simulink model "System_Model_discrete"  (Simulink 7.6)
settings: Solver=ode15s  StartTime=0.0  StopTime=3  RelTol=1e-3
undefined symbols (not defined in the file): C, dd, denhigh, denlow, DiscIntNeverNeededParam, F, G, g, H, K, L0, m, magnitude, nd, Nu, numhigh, numlow, Nx, Q, R, Ts, u0, x01, x02, x03
libraries: fl_lib x18, nesl_utility x6, simulink x5, elec_lib x1
CloseFcn:
  | rtwprivate ssgencode ModelCloseRequest System_Model1
settings Model: Creator=Fodi  LastModifiedBy=Fodi

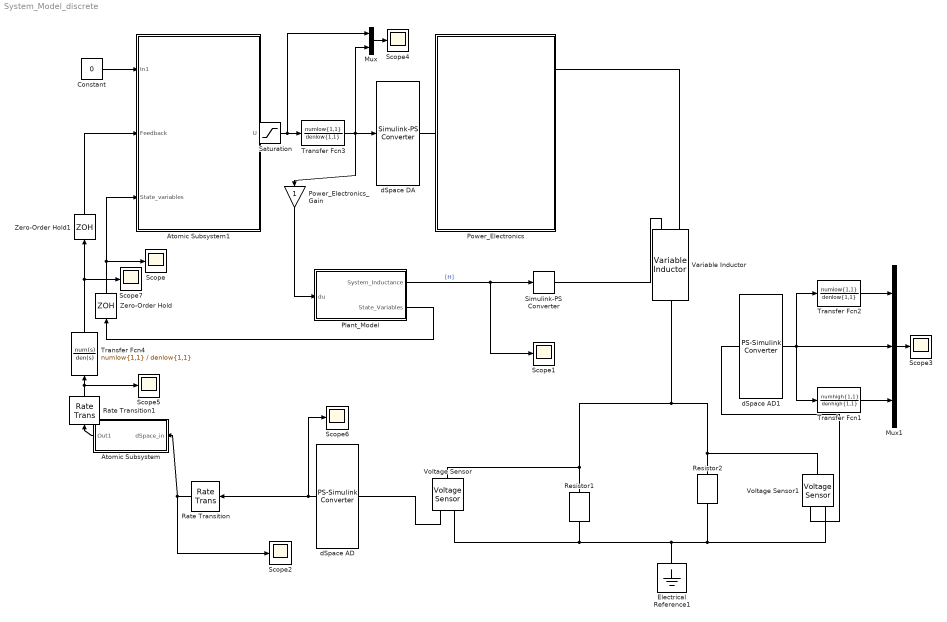
== system System_Model_discrete ==
  Atomic Subsystem : Subsystem  TreatAsAtomicUnit=on
  Atomic Subsystem1 : Subsystem  TreatAsAtomicUnit=on  SystemSampleTime=Ts
  Constant : Constant  Value=0
  Electrical Reference1 : fl_lib/Electrical/Electrical Elements/Electrical Reference  DialogController=NetworkEngine.DynNeDlgSource  SystemSampleTime=-1  i_Log=off  LocalVarNames=|i  LocalVarDescs=|i  LocalVarLogging=0
  Mux : Mux  Inputs=2
  Mux1 : Mux  Inputs=3
  Plant_Model : Subsystem
  Power_Electronics : Subsystem
  Power_Electronics_Gain : Gain
  Rate Transition : RateTransition  OutPortSampleTime=0.0001
  Rate Transition1 : RateTransition  OutPortSampleTime=0.0001
  Resistor1 : fl_lib/Electrical/Electrical Elements/Resistor  DialogController=NetworkEngine.DynNeDlgSource  SystemSampleTime=-1  R=100 Ohm  i_Log=off  v_Log=off  LocalVarNames=|i|v  LocalVarDescs=|i|v  LocalVarLogging=[0 0]
  Resistor2 : fl_lib/Electrical/Electrical Elements/Resistor  DialogController=NetworkEngine.DynNeDlgSource  SystemSampleTime=-1  R=100 Ohm  i_Log=off  v_Log=off  LocalVarNames=|i|v  LocalVarDescs=|i|v  LocalVarLogging=[0 0]
  Saturation : Saturate  UpperLimit=3000  LowerLimit=-u0
  Scope{,1..7} (8 alike) : Scope
      Scope settings: YMin=-3e-006  YMax=1.75e-006  SaveName=ScopeData7
      Scope1 settings: YMin=0.266286  YMax=0.266289  SaveName=ScopeData5
      Scope2 settings: YMin=0.266286  YMax=0.266289  SaveName=ScopeData4
      Scope3 settings: YMin=-2.5  YMax=50  SaveName=ScopeData10
      Scope4 settings: YMin=0.1375  YMax=0.142  SaveName=ScopeData6
      Scope5 settings: YMin=0.266286  YMax=0.266289  SaveName=ScopeData11
      Scope6 settings: TimeRange=0.0315055374939181  YMin=-25.11022062082716  YMax=-22.69283608820259  SaveName=ScopeData12
      Scope7 settings: YMin=0.266286  YMax=0.266289  SaveName=ScopeData20
  Simulink-PS Converter : nesl_utility/Simulink-PS Converter  DialogController=NetworkEngine.DynNeUtilDlgSource  SystemSampleTime=-1  PhysicalDomain=network_engine_domain  LeftPortType=input  RightPortType=output  SubClassName=ps_input  Unit=1  AffineConversion=off  InputFilterTimeConstant=.001  UdotUserProvided=0
  Transfer Fcn1 : TransferFcn  Numerator=numhigh{1,1}  Denominator=denhigh{1,1}
  Transfer Fcn2 : TransferFcn  Numerator=numlow{1,1}  Denominator=denlow{1,1}
  Transfer Fcn3 : TransferFcn  Numerator=numlow{1,1}  Denominator=denlow{1,1}
  Transfer Fcn4 : TransferFcn  Numerator=numlow{1,1}  Denominator=denlow{1,1}
  Variable Inductor : elec_lib/Passive Devices/Variable Inductor  DialogController=NetworkEngine.DynNeDlgSource  SystemSampleTime=-1  prm=2  Lmin=1e-6 H  g=1e-9 1/Ohm  i0=0 A  phi0=0 Wb  LocalVarLogging=[]
  Voltage Sensor : fl_lib/Electrical/Electrical Sensors/Voltage Sensor  DialogController=NetworkEngine.DynNeDlgSource  SystemSampleTime=-1  i1_Log=off  v1_Log=off  LocalVarNames=|i1|v1  LocalVarDescs=|i1|v1  LocalVarLogging=[0 0]
  Voltage Sensor1 : fl_lib/Electrical/Electrical Sensors/Voltage Sensor  DialogController=NetworkEngine.DynNeDlgSource  SystemSampleTime=-1  i1_Log=off  v1_Log=off  LocalVarNames=|i1|v1  LocalVarDescs=|i1|v1  LocalVarLogging=[0 0]
  Zero-Order Hold : ZeroOrderHold  SampleTime=Ts
  Zero-Order Hold1 : ZeroOrderHold  SampleTime=0.001
  dSpace AD : nesl_utility/PS-Simulink Converter  DialogController=NetworkEngine.DynNeUtilDlgSource  SystemSampleTime=-1  PhysicalDomain=network_engine_domain  LeftPortType=input  RightPortType=output  SubClassName=ps_output  Unit=1  AffineConversion=off
  dSpace AD1 : nesl_utility/PS-Simulink Converter  DialogController=NetworkEngine.DynNeUtilDlgSource  SystemSampleTime=-1  PhysicalDomain=network_engine_domain  LeftPortType=input  RightPortType=output  SubClassName=ps_output  Unit=1  AffineConversion=off
  dSpace DA : nesl_utility/Simulink-PS Converter  DialogController=NetworkEngine.DynNeUtilDlgSource  SystemSampleTime=-1  PhysicalDomain=network_engine_domain  LeftPortType=input  RightPortType=output  SubClassName=ps_input  Unit=1  AffineConversion=off  InputFilterTimeConstant=.001  UdotUserProvided=0
  wires:
  Plant_Model/1(System_Inductance) -> Scope1/1, Simulink-PS Converter/1  "[H]"
  Atomic Subsystem1/1(U) -> Saturation/1
  Power_Electronics_Gain/1 -> Plant_Model/1(du)
  Plant_Model/2(State_Variables) -> Zero-Order Hold/1
  Constant/1 -> Atomic Subsystem1/1(In1)
  dSpace AD/1 -> Rate Transition/1, Scope6/1
  Zero-Order Hold/1 -> Scope/1, Atomic Subsystem1/3(State_variables)
  Rate Transition/1 -> Atomic Subsystem/1(dSpace_in), Scope2/1
  Atomic Subsystem/1(Out1) -> Rate Transition1/1
  Zero-Order Hold1/1 -> Atomic Subsystem1/2(Feedback)
  Saturation/1 -> Mux/1, Transfer Fcn3/1
  Mux/1 -> Scope4/1
  dSpace AD1/1 -> Mux1/2, Transfer Fcn2/1, Transfer Fcn1/1
  Transfer Fcn2/1 -> Mux1/1
  Transfer Fcn1/1 -> Mux1/3
  Mux1/1 -> Scope3/1
  Transfer Fcn3/1 -> dSpace DA/1, Power_Electronics_Gain/1, Mux/2
  Transfer Fcn4/1 -> Zero-Order Hold1/1, Scope7/1
  Rate Transition1/1 -> Scope5/1, Transfer Fcn4/1
  connections:
  dSpace DA/RConn1 -- Power_Electronics/LConn1
  Voltage Sensor/RConn2 -- Resistor2/RConn1 -- Voltage Sensor1/RConn2 -- Electrical Reference1/LConn1 -- Resistor1/RConn1
  Voltage Sensor/RConn1 -- dSpace AD/LConn1
  Simulink-PS Converter/RConn1 -- Variable Inductor/LConn1
  Power_Electronics/RConn1 -- Variable Inductor/LConn2
  Voltage Sensor1/RConn1 -- dSpace AD1/LConn1
  Variable Inductor/RConn1 -- Resistor2/LConn1 -- Voltage Sensor1/LConn1 -- Resistor1/LConn1 -- Voltage Sensor/LConn1

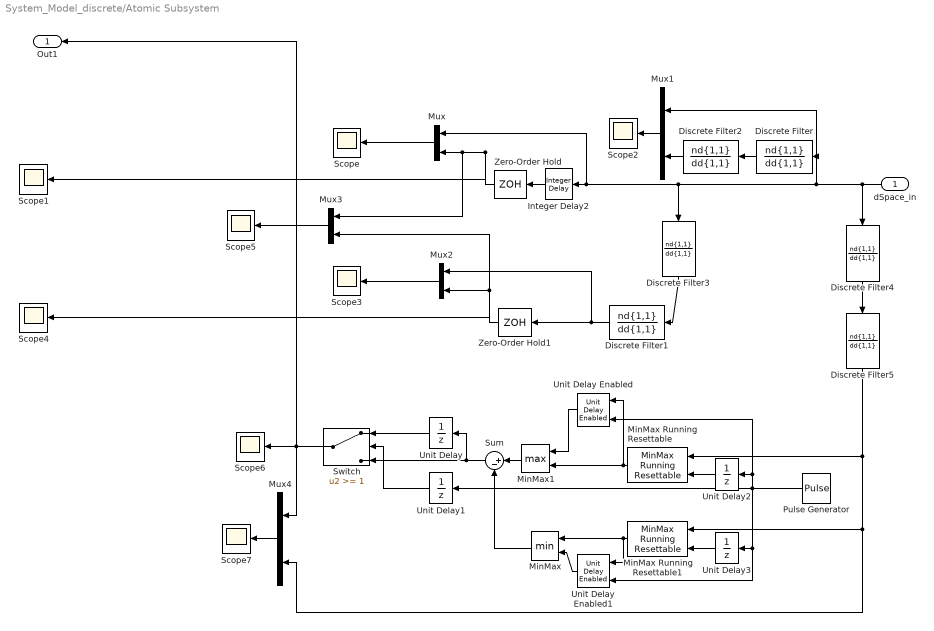
== system System_Model_discrete/Atomic Subsystem ==
  dSpace_in : Inport
  Discrete Filter{,1..5} (6 alike) : DiscreteFilter  Numerator=nd{1,1}  Denominator=dd{1,1}
  Integer Delay2 : simulink/Discrete/Integer Delay  NumDelays=1  vinit=0.0  samptime=-1
  MinMax : MinMax  Inputs=2
  MinMax Running Resettable : simulink/Math Operations/MinMax Running Resettable  SystemSampleTime=-1  Function=max  vinit=0.0
  MinMax Running Resettable1 : simulink/Math Operations/MinMax Running Resettable  SystemSampleTime=-1  Function=min  vinit=0.0
  MinMax1 : MinMax  Function=max  Inputs=2
  Mux{,1..4} (5 alike) : Mux  Inputs=2
  Pulse Generator : DiscretePulseGenerator  Period=10  SampleTime=-1
  Scope{,1..7} (8 alike) : Scope
      Scope settings: TimeRange=7  YMin=-9.407420347240764e-006  YMax=1.255471123145118e-005  SaveName=ScopeData2
      Scope1 settings: TimeRange=7  YMin=-9.407420347240764e-006  YMax=1.255471123145118e-005  SaveName=ScopeData13
      Scope2 settings: TimeRange=7  YMin=-9.407420347240764e-006  YMax=1.255471123145118e-005  SaveName=ScopeData14
      Scope3 settings: TimeRange=7  YMin=-9.407420347240764e-006  YMax=1.255471123145118e-005  SaveName=ScopeData16
      Scope4 settings: TimeRange=7  YMin=-9.407420347240764e-006  YMax=1.255471123145118e-005  SaveName=ScopeData18
      Scope5 settings: TimeRange=7  YMin=-9.407420347240764e-006  YMax=1.255471123145118e-005  SaveName=ScopeData19
      Scope6 settings: TimeRange=3  YMin=0  YMax=1200  SaveName=ScopeData15
      Scope7 settings: TimeRange=7  YMin=-9.407420347240764e-006  YMax=1.255471123145118e-005  SaveName=ScopeData21
  Sum : Sum  Inputs=|+-
  Switch : Switch  Threshold=1
  Unit Delay{,1..3} (4 alike) : UnitDelay  SampleTime=-1
  Unit Delay Enabled : simulink/Additional Math & Discrete/Additional Discrete/Unit Delay Enabled  SystemSampleTime=-1  vinit=0.0  tsamp=-1
  Unit Delay Enabled1 : simulink/Additional Math & Discrete/Additional Discrete/Unit Delay Enabled  SystemSampleTime=-1  vinit=0.0  tsamp=-1
  Zero-Order Hold : ZeroOrderHold  SampleTime=1/1000
  Zero-Order Hold1 : ZeroOrderHold  SampleTime=1/1000
  Out1 : Outport
  wires:
  Zero-Order Hold/1 -> Scope1/1, Mux/2, Mux3/1
  Mux/1 -> Scope/1
  dSpace_in/1 -> Discrete Filter/1, Mux1/1, Mux/1, Integer Delay2/1, Discrete Filter3/1, Discrete Filter4/1
  Integer Delay2/1 -> Zero-Order Hold/1
  Mux1/1 -> Scope2/1
  Discrete Filter/1 -> Discrete Filter2/1
  Zero-Order Hold1/1 -> Scope4/1, Mux2/2, Mux3/2
  Mux2/1 -> Scope3/1
  Discrete Filter1/1 -> Mux2/1, Zero-Order Hold1/1
  Mux3/1 -> Scope5/1
  Discrete Filter2/1 -> Mux1/2
  Discrete Filter3/1 -> Discrete Filter1/1
  MinMax Running Resettable1/1 -> MinMax/1, Unit Delay Enabled1/1
  Pulse Generator/1 -> Unit Delay Enabled/2, Unit Delay2/1, Unit Delay Enabled1/2, Unit Delay3/1, Unit Delay1/1
  Switch/1 -> Scope6/1, Out1/1, Mux4/1
  Sum/1 -> Switch/3, Unit Delay/1
  Unit Delay/1 -> Switch/1
  Mux4/1 -> Scope7/1
  Discrete Filter4/1 -> Discrete Filter5/1
  Discrete Filter5/1 -> MinMax Running Resettable/1, MinMax Running Resettable1/1, Mux4/2
  MinMax/1 -> Sum/2
  MinMax1/1 -> Sum/1
  MinMax Running Resettable/1 -> MinMax1/2, Unit Delay Enabled/1
  Unit Delay Enabled/1 -> MinMax1/1
  Unit Delay Enabled1/1 -> MinMax/2
  Unit Delay1/1 -> Switch/2
  Unit Delay2/1 -> MinMax Running Resettable/2
  Unit Delay3/1 -> MinMax Running Resettable1/2

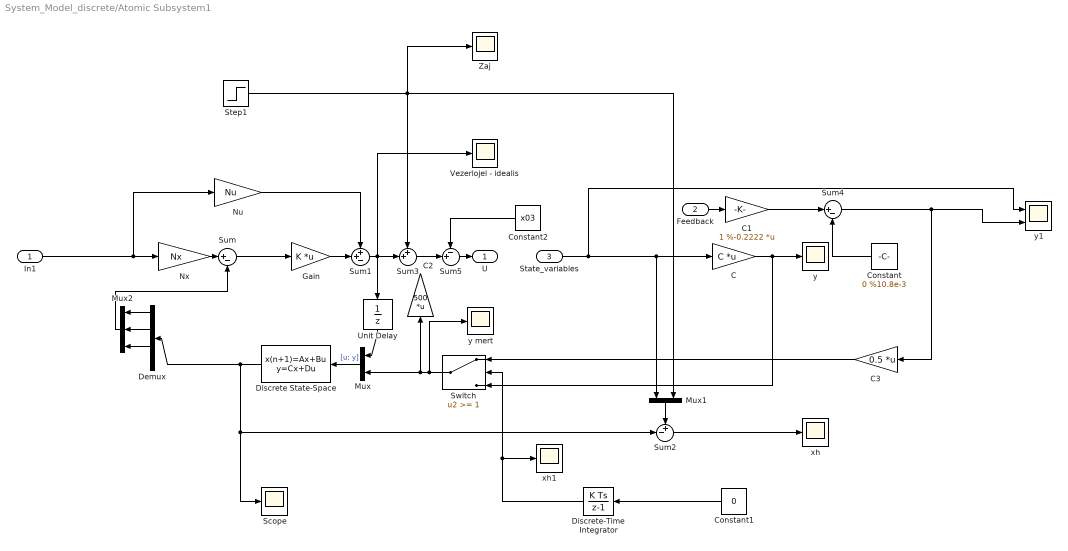
== system System_Model_discrete/Atomic Subsystem1 ==
  In1 : Inport
  Feedback : Inport  Port=2
  State_variables : Inport  Port=3
  C : Gain  Gain=C  Multiplication=Matrix(K*u)
  C1 : Gain  Gain=1 %-0.2222  Multiplication=Matrix(K*u)
  C2 : Gain  Gain=500  Multiplication=Matrix(K*u)
  C3 : Gain  Gain=0.5  Multiplication=Matrix(K*u)
  Constant : Constant  Value=0 %10.8e-3
  Constant1 : Constant  Value=0
  Constant2 : Constant  Value=x03
  Demux : Demux
  Discrete State-Space : DiscreteStateSpace  A=F  B=[H G]  C=eye(size(F))  D=zeros(size(F,1),size([H G],2))  SampleTime=Ts
  Discrete-Time Integrator : DiscreteIntegrator  gainval=1  SampleTime=-1  ICPrevOutput=DiscIntNeverNeededParam  ICPrevScaledInput=DiscIntNeverNeededParam
  Gain : Gain  Gain=K  Multiplication=Matrix(K*u)
  Mux : Mux  Inputs=2
  Mux1 : Mux  Inputs=2
  Mux2 : Mux  Inputs=3
  Nu : Gain  Gain=Nu
  Nx : Gain  Gain=Nx
  Scope : Scope
      settings: SaveName=xb
  Step1 : Step  Time=2  After=0  SampleTime=Ts
  Sum : Sum  Inputs=|+-
  Sum1 : Sum  Inputs=++-
  Sum2 : Sum  Inputs=+-|
  Sum3 : Sum  Inputs=++|
  Sum4 : Sum  Inputs=|+-
  Sum5 : Sum  Inputs=-+|
  Switch : Switch  Threshold=1
  Unit Delay : UnitDelay  SampleTime=-1
  Vezerlojel - idealis : Scope
      settings: TimeRange=10  YMin=-1  YMax=3  SaveName=u
  Zaj : Scope
      settings: SaveName=ScopeData8
  xh : Scope
      settings: TimeRange=10  YMin=-0.02  YMax=0.12  SaveName=ScopeData9
  xh1 : Scope
      settings: TimeRange=10  YMin=-0.02  YMax=0.12  SaveName=ScopeData17
  y : Scope
      settings: TimeRange=10  YMin=0  YMax=0.0025  SaveName=y
  y mert : Scope
      settings: TimeRange=5  YMin=0  YMax=0.003  SaveName=ym
  y1 : Scope  NumInputPorts=2
      settings: TimeRange=1.5  YMin=-0.03~0  YMax=0.11~350  SaveName=y1
  U : Outport
  wires:
  In1/1 -> Nx/1, Nu/1
  Nx/1 -> Sum/1
  Nu/1 -> Sum1/1
  Gain/1 -> Sum1/2
  Sum/1 -> Gain/1
  Sum1/1 -> Sum3/2, Vezerlojel - idealis/1, Unit Delay/1
  State_variables/1 -> C/1, Mux1/1, y1/1
  Mux/1 -> Discrete State-Space/1  "[u; y]"
  Step1/1 -> Sum3/1, Mux1/2, Zaj/1
  Mux1/1 -> Sum2/1
  Mux2/1 -> Sum/2
  Demux/1 -> Mux2/1
  Demux/2 -> Mux2/2
  Demux/3 -> Mux2/3
  Sum2/1 -> xh/1
  C/1 -> y/1, Switch/3
  Discrete State-Space/1 -> Demux/1, Sum2/2, Scope/1
  Unit Delay/1 -> Mux/1
  Feedback/1 -> C1/1
  Sum4/1 -> y1/2, C3/1
  Constant/1 -> Sum4/2
  Switch/1 -> y mert/1, Mux/2, C2/1
  C1/1 -> Sum4/1
  Discrete-Time Integrator/1 -> Switch/2, xh1/1
  Constant1/1 -> Discrete-Time Integrator/1
  Constant2/1 -> Sum5/1
  Sum5/1 -> U/1
  Sum3/1 -> Sum5/2
  C3/1 -> Switch/1

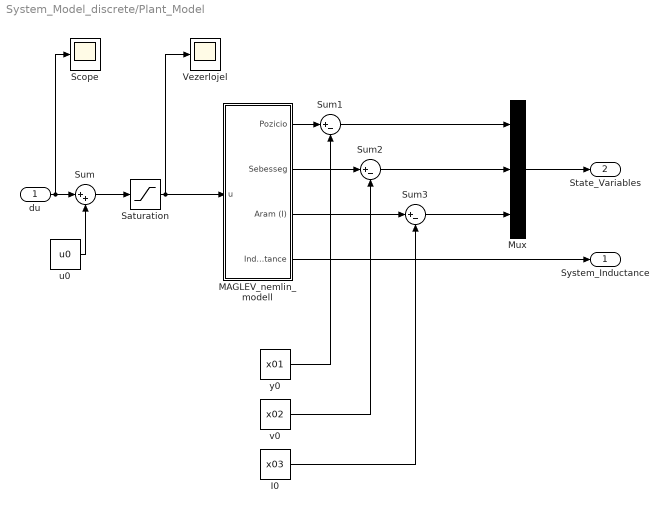
== system System_Model_discrete/Plant_Model ==
  du : Inport
  I0 : Constant  Value=x03
  MAGLEV_nemlin_modell : Subsystem
  Mux : Mux  Inputs=3
  Saturation : Saturate  UpperLimit=30  LowerLimit=-30
  Scope : Scope
  Sum : Sum  Inputs=|++
  Sum1 : Sum  Inputs=|+-
  Sum2 : Sum  Inputs=|+-
  Sum3 : Sum  Inputs=|+-
  Vezerlojel : Scope
      settings: TimeRange=10  YMin=11  YMax=16
  u0 : Constant  Value=u0
  v0 : Constant  Value=x02
  y0 : Constant  Value=x01
  System_Inductance : Outport
  State_Variables : Outport  Port=2
  wires:
  y0/1 -> Sum1/2
  v0/1 -> Sum2/2
  I0/1 -> Sum3/2
  MAGLEV_nemlin_modell/3(Aram (I)) -> Sum3/1
  Sum3/1 -> Mux/3
  Sum2/1 -> Mux/2
  Sum1/1 -> Mux/1
  u0/1 -> Sum/2
  Mux/1 -> State_Variables/1
  MAGLEV_nemlin_modell/2(Sebesseg) -> Sum2/1
  MAGLEV_nemlin_modell/1(Pozicio) -> Sum1/1
  du/1 -> Scope/1, Sum/1
  Sum/1 -> Saturation/1
  Saturation/1 -> MAGLEV_nemlin_modell/1(u), Vezerlojel/1
  MAGLEV_nemlin_modell/4(Inductance) -> System_Inductance/1

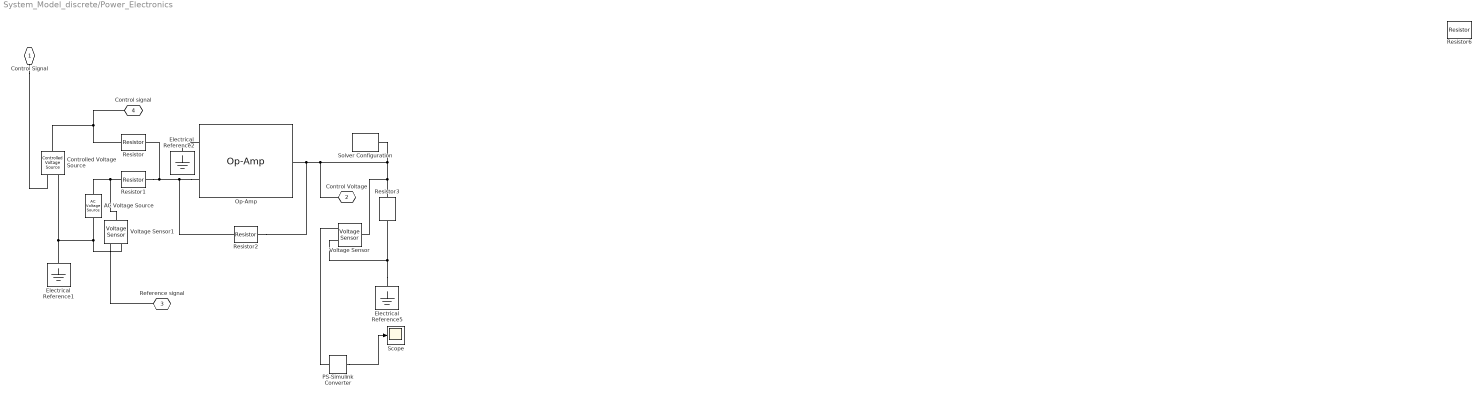
== system System_Model_discrete/Power_Electronics ==
  AC Voltage Source : fl_lib/Electrical/Electrical Sources/AC Voltage Source  DialogController=NetworkEngine.DynNeDlgSource  SystemSampleTime=-1  amp=50 mV  shift=90 deg  omega=1000 Hz  i_Log=off  v_Log=off  LocalVarNames=|i|v  LocalVarDescs=|i|v  LocalVarLogging=[0 0]
  Controlled Voltage Source : fl_lib/Electrical/Electrical Sources/Controlled Voltage Source  DialogController=NetworkEngine.DynNeDlgSource  SystemSampleTime=-1  i_Log=off  v_Log=off  LocalVarNames=|i|v  LocalVarDescs=|i|v  LocalVarLogging=[0 0]
  Electrical Reference1 : fl_lib/Electrical/Electrical Elements/Electrical Reference  DialogController=NetworkEngine.DynNeDlgSource  SystemSampleTime=-1  i_Log=off  LocalVarNames=|i  LocalVarDescs=|i  LocalVarLogging=0
  Electrical Reference2 : fl_lib/Electrical/Electrical Elements/Electrical Reference  DialogController=NetworkEngine.DynNeDlgSource  SystemSampleTime=-1  i_Log=off  LocalVarNames=|i  LocalVarDescs=|i  LocalVarLogging=0
  Electrical Reference5 : fl_lib/Electrical/Electrical Elements/Electrical Reference  DialogController=NetworkEngine.DynNeDlgSource  SystemSampleTime=-1  i_Log=off  LocalVarNames=|i  LocalVarDescs=|i  LocalVarLogging=0
  Op-Amp : fl_lib/Electrical/Electrical Elements/Op-Amp  DialogController=NetworkEngine.DynNeDlgSource  SystemSampleTime=-1  i1_Log=off  v1_Log=off  outI_Log=off  LocalVarNames=|i1|v1|outI  LocalVarDescs=|i1|v1|outI  LocalVarLogging=[0 0 0]
  PS-Simulink Converter : nesl_utility/PS-Simulink Converter  DialogController=NetworkEngine.DynNeUtilDlgSource  SystemSampleTime=-1  PhysicalDomain=network_engine_domain  LeftPortType=input  RightPortType=output  SubClassName=ps_output  Unit=1  AffineConversion=off
  Resistor : fl_lib/Electrical/Electrical Elements/Resistor  DialogController=NetworkEngine.DynNeDlgSource  SystemSampleTime=-1  R=1 kOhm  i_Log=off  v_Log=off  LocalVarNames=|i|v  LocalVarDescs=|i|v  LocalVarLogging=[0 0]
  Resistor1 : fl_lib/Electrical/Electrical Elements/Resistor  DialogController=NetworkEngine.DynNeDlgSource  SystemSampleTime=-1  R=1 kOhm  i_Log=off  v_Log=off  LocalVarNames=|i|v  LocalVarDescs=|i|v  LocalVarLogging=[0 0]
  Resistor2 : fl_lib/Electrical/Electrical Elements/Resistor  DialogController=NetworkEngine.DynNeDlgSource  SystemSampleTime=-1  R=100 kOhm  i_Log=off  v_Log=off  LocalVarNames=|i|v  LocalVarDescs=|i|v  LocalVarLogging=[0 0]
  Resistor3 : fl_lib/Electrical/Electrical Elements/Resistor  DialogController=NetworkEngine.DynNeDlgSource  SystemSampleTime=-1  R=100 kOhm  i_Log=off  v_Log=off  LocalVarNames=|i|v  LocalVarDescs=|i|v  LocalVarLogging=[0 0]
  Resistor6 : fl_lib/Electrical/Electrical Elements/Resistor  DialogController=NetworkEngine.DynNeDlgSource  SystemSampleTime=-1  R=1 kOhm  i_Log=off  v_Log=off  LocalVarNames=|i|v  LocalVarDescs=|i|v  LocalVarLogging=[0 0]
  Scope : Scope
      settings: SaveName=ScopeData3
  Solver Configuration : nesl_utility/Solver Configuration  DialogController=NetworkEngine.DynNeUtilDlgSource  SystemSampleTime=-1  PhysicalDomain=network_engine_domain  LeftPortType=input  RightPortType=generic  SubClassName=solver  Accelerate=off  Profile=off  ResidualTolerance=1e-9  MaxNonlinIter=3  MaxModeIter=2  DoFixedCost=off  UseLocalSampling=off  DoDC=off  LinearAlgebra=Sparse  LocalSolverSampleTime=.001  LocalSolverChoice=NE_BACKWARD_EULER_ADVANCER  UseLocalSolver=off
  Voltage Sensor : fl_lib/Electrical/Electrical Sensors/Voltage Sensor  DialogController=NetworkEngine.DynNeDlgSource  SystemSampleTime=-1  i1_Log=off  v1_Log=off  LocalVarNames=|i1|v1  LocalVarDescs=|i1|v1  LocalVarLogging=[0 0]
  Voltage Sensor1 : fl_lib/Electrical/Electrical Sensors/Voltage Sensor  DialogController=NetworkEngine.DynNeDlgSource  SystemSampleTime=-1  i1_Log=off  v1_Log=off  LocalVarNames=|i1|v1  LocalVarDescs=|i1|v1  LocalVarLogging=[0 0]
  Control Signal : PMIOPort  Tag=PMCPort  Port=1  Side=Left
  Control Voltage : PMIOPort  Tag=PMCPort  Port=2  Side=Right
  Reference signal : PMIOPort  Tag=PMCPort  Port=3  Side=Right
  Control signal : PMIOPort  Tag=PMCPort  Port=4  Side=Right
  wires:
  PS-Simulink Converter/1 -> Scope/1
  connections:
  Op-Amp/LConn2 -- Resistor2/LConn1 -- Resistor/RConn1 -- Resistor1/RConn1
  Solver Configuration/RConn1 -- Resistor3/LConn1 -- Voltage Sensor/LConn1 -- Control Voltage/RConn1 -- Op-Amp/RConn1 -- Resistor2/RConn1
  Electrical Reference5/LConn1 -- Voltage Sensor/RConn2 -- Resistor3/RConn1
  Controlled Voltage Source/LConn1 -- Resistor/LConn1 -- Control signal/RConn1
  AC Voltage Source/RConn1 -- Voltage Sensor1/RConn2 -- Controlled Voltage Source/RConn2 -- Electrical Reference1/LConn1
  AC Voltage Source/LConn1 -- Resistor1/LConn1 -- Voltage Sensor1/LConn1
  Op-Amp/LConn1 -- Electrical Reference2/LConn1
  Voltage Sensor/RConn1 -- PS-Simulink Converter/LConn1
  Voltage Sensor1/RConn1 -- Reference signal/RConn1
  Control Signal/RConn1 -- Controlled Voltage Source/RConn1

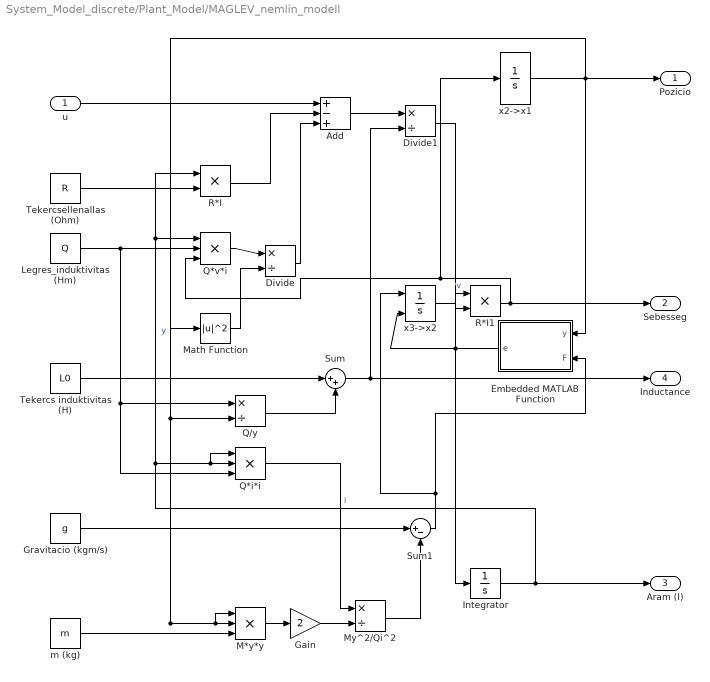
== system System_Model_discrete/Plant_Model/MAGLEV_nemlin_modell ==
  u : Inport  Tag=v
  Add : Sum  Inputs=+-+
  Divide : Product  Inputs=*/
  Divide1 : Product  Inputs=*/
  Embedded MATLAB Function : Stateflow chart  TreatAsAtomicUnit=on
  Gain : Gain  Gain=2
  Gravitacio (kgm/s) : Constant  Value=g
  Integrator : Integrator  LimitOutput=on  LowerSaturationLimit=0  ContinuousStateAttributes='current'
  Legres_induktivitas (Hm) : Constant  Value=Q
  M*y*y : Product  Inputs=3  RndMeth=Zero
  Math Function : Math  Operator=magnitude^2  SaturateOnIntegerOverflow=on
  My^2/Qi^2 : Product  Inputs=*/
  Q*i*i : Product  Inputs=3  RndMeth=Zero
  Q*v*i : Product  Inputs=3  RndMeth=Zero
  Q/y : Product  Inputs=*/
  R*I : Product  RndMeth=Zero
  R*I1 : Product  RndMeth=Zero
  Sum : Sum  Inputs=|++
  Sum1 : Sum  Inputs=|+-
  Tekercs induktivitas (H) : Constant  Value=L0
  Tekercsellenallas (Ohm) : Constant  Value=R
  m (kg) : Constant  Value=m
  x2->x1 : Integrator  InitialCondition=x01+0.001  LimitOutput=on  LowerSaturationLimit=0.001  ContinuousStateAttributes='position'
  x3->x2 : Integrator  ExternalReset=rising  ContinuousStateAttributes='speed'
  Pozicio : Outport
  Sebesseg : Outport  Port=2
  Aram (I) : Outport  Port=3
  Inductance : Outport  Port=4
  wires:
  x2->x1/1 -> Q/y/2, Math Function/1, M*y*y/2, M*y*y/1, Pozicio/1, Embedded MATLAB Function/1(y)  "y"
  Gravitacio (kgm/s)/1 -> Sum1/1
  My^2/Qi^2/1 -> Sum1/2
  Gain/1 -> My^2/Qi^2/2
  M*y*y/1 -> Gain/1
  Sum/1 -> Divide1/2, Inductance/1
  Tekercs induktivitas (H)/1 -> Sum/1
  Q/y/1 -> Sum/2
  Math Function/1 -> Divide/2
  Divide/1 -> Add/3
  Q*v*i/1 -> Divide/1
  R*I/1 -> Add/2
  Divide1/1 -> Integrator/1
  Add/1 -> Divide1/1
  u/1 -> Add/1
  m (kg)/1 -> M*y*y/3
  Legres_induktivitas (Hm)/1 -> Q*v*i/2, Q/y/1, Q*i*i/3
  Tekercsellenallas (Ohm)/1 -> R*I/2
  Q*i*i/1 -> My^2/Qi^2/1
  Integrator/1 -> Aram (I)/1, Q*i*i/2, Q*i*i/1, Q*v*i/1, R*I/1  "i"
  Sum1/1 -> x3->x2/1, Embedded MATLAB Function/2(F)
  Embedded MATLAB Function/1(e) -> x3->x2/2, R*I1/2
  R*I1/1 -> Q*v*i/3, x2->x1/1, Sebesseg/1
  x3->x2/1 -> R*I1/1  "v"

== matlab function Plant_Model/MAGLEV_nemlin_modell/Embedded MATLAB Function ==
  data: y input double; F input double; e output double
function e = fcn(y, F)
%#eml

if (F<=0 && y == 0.001)
    e=0;
else
    e=1;
end

end
